simulink model "BGR300"  (R2023a)
settings: Solver=VariableStepAuto  StartTime=0.0  StopTime=5  RelTol=1e-3
values from neighbouring files (symbols this model uses):
  Jb = Jb + (31599185/1000/1000000)*rb*rb    (= 5.14719290283e-06)    [parametres.m]
  Kb = 20.8/1000    (= 0.0208)    [parametres.m]
  Lb = 0.186e-3    (= 0.000186)    [parametres.m]
  rb = 1/92.7    (= 0.0107874865156)    [parametres.m]
  Rb = 1.53    [parametres.m]
settings Model: Creator=xpess  LastModifiedBy=xpess

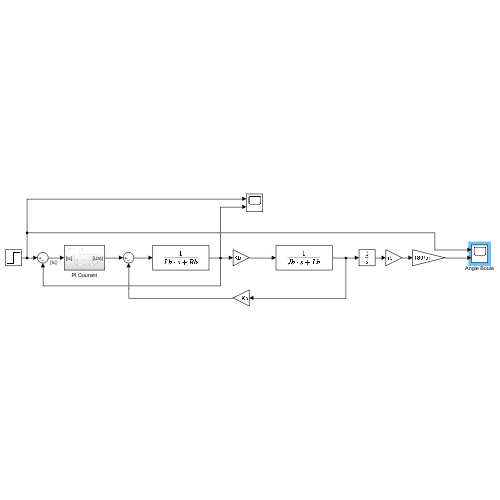
[thumbnail: Simulink's stored preview of the top-level diagram]
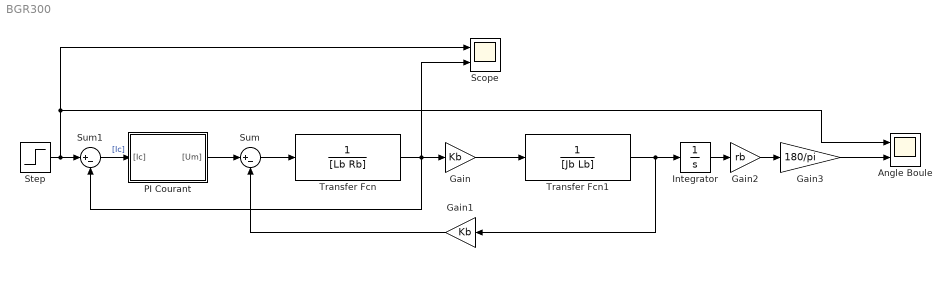
== system BGR300 ==
  Angle Boule : Scope  NumInputPorts=2
  Gain : Gain  Gain=Kb
  Gain1 : Gain  Gain=Kb
  Gain2 : Gain  Gain=rb
  Gain3 : Gain  Gain=180/pi
  Integrator : Integrator
  PI Courant : Subsystem
  Scope : Scope  NumInputPorts=2
  Step : Step  SampleTime=0
  Sum : Sum  Inputs=|+-
  Sum1 : Sum  Inputs=|+-
  Transfer Fcn : TransferFcn  Denominator=[Lb Rb]
  Transfer Fcn1 : TransferFcn  Denominator=[Jb Lb]
  wires:
  Transfer Fcn/1 -> Scope/2, Sum1/2, Gain/1
  Gain/1 -> Transfer Fcn1/1
  Transfer Fcn1/1 -> Gain1/1, Integrator/1
  Sum/1 -> Transfer Fcn/1
  Gain1/1 -> Sum/2
  Integrator/1 -> Gain2/1
  Gain2/1 -> Gain3/1
  Step/1 -> Scope/1, Angle Boule/1, Sum1/1
  Gain3/1 -> Angle Boule/2
  Sum1/1 -> PI Courant/1("[Ic]")  "[Ic]"
  PI Courant/1("[Um]") -> Sum/1

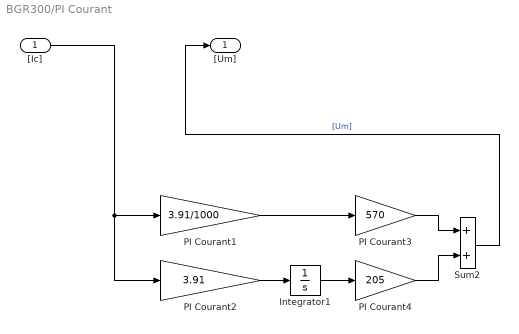
== system BGR300/PI Courant ==
  "[Ic]" : Inport
  Integrator1 : Integrator
  PI Courant1 : Gain  Gain=3.91/1000
  PI Courant2 : Gain  Gain=3.91
  PI Courant3 : Gain  Gain=570
  PI Courant4 : Gain  Gain=205
  Sum2 : Sum
  "[Um]" : Outport
  wires:
  "[Ic]"/1 -> PI Courant2/1, PI Courant1/1
  PI Courant4/1 -> Sum2/2
  Integrator1/1 -> PI Courant4/1
  PI Courant1/1 -> PI Courant3/1
  PI Courant3/1 -> Sum2/1
  Sum2/1 -> "[Um]"/1  "[Um]"
  PI Courant2/1 -> Integrator1/1
